simulink model "q5_tf"  (R2017b)
settings: Solver=VariableStepAuto  StartTime=0.0  StopTime=10.0  RelTol=1e-3
settings Model: Creator=nadav  LastModifiedBy=nadav

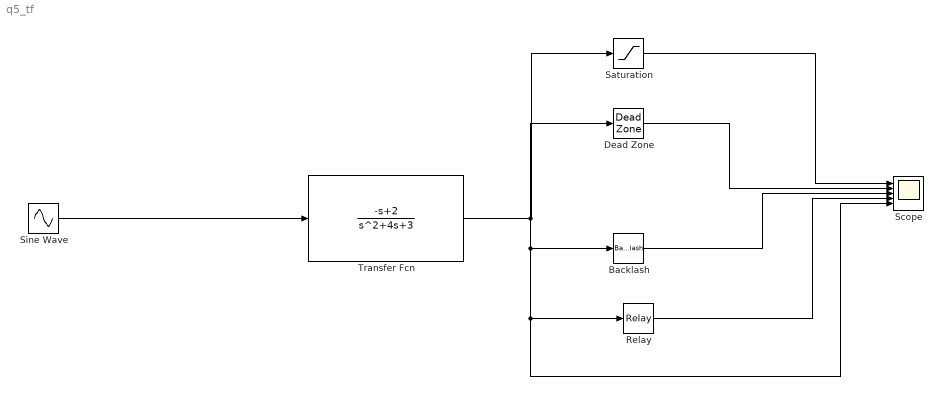
== system q5_tf ==
  Backlash : Backlash  BacklashWidth=0.1
  Dead Zone : DeadZone  LowerValue=-0.1  UpperValue=0.1  SaturateOnIntegerOverflow=on
  Relay : Relay  OnOutputValue=0.2  OffOutputValue=-0.2
  Saturation : Saturate  UpperLimit=0.1  LowerLimit=-0.1
  Scope : Scope  NumInputPorts=5
  Sine Wave : Sin  Frequency=5  SampleTime=0
  Transfer Fcn : TransferFcn  Numerator=[-1 2]  Denominator=[1 4 3]
  wires:
  Sine Wave/1 -> Transfer Fcn/1
  Transfer Fcn/1 -> Dead Zone/1, Scope/5, Relay/1, Backlash/1, Saturation/1
  Relay/1 -> Scope/4
  Backlash/1 -> Scope/3
  Saturation/1 -> Scope/1
  Dead Zone/1 -> Scope/2
